simulink model "untitled1"  (R2023b)
settings: Solver=ode23  StartTime=0.0  StopTime=10.0  RelTol=1e-3
settings Model: Creator=ray  LastModifiedBy=ray

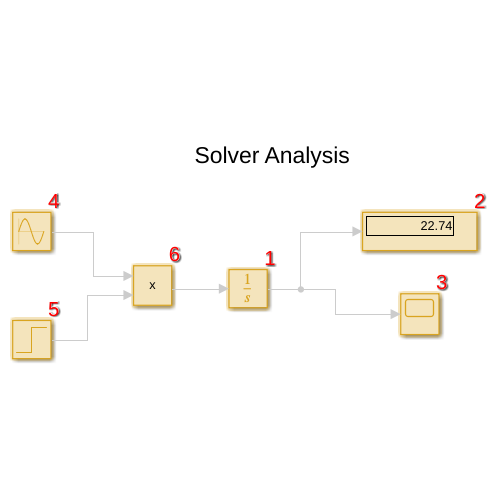
[thumbnail: Simulink's stored preview of the top-level diagram]
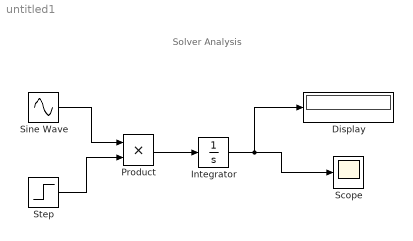
== system untitled1 ==
  note: Solver Analysis
  Display : Display
  Integrator : Integrator
  Product : Product
  Scope : Scope
  Sine Wave : Sin  Amplitude=5  Frequency=0.1  SampleTime=0
  Step : Step  SampleTime=0
  wires:
  Step/1 -> Product/2
  Sine Wave/1 -> Product/1
  Product/1 -> Integrator/1
  Integrator/1 -> Display/1, Scope/1
